simulink model "Ident_friccion_step2_GB3"  (Simulink 6.6)
settings: Solver=ode4  StartTime=0.0  StopTime=1000  RelTol=1e-6
PreLoadFcn:
  | inicializacion_step2
StopFcn:
  | saveDATA_Ident_friccion_STEP2_GB
values from neighbouring files (symbols this model uses):
  k5_id = 0.921382714286    [Valores_identificados_STEP1.mat]
  kb_id = 2.2683494    [Valores_identificados_STEP1.mat]
  Ki1 = 0.0195    [inicializacion_step2.m]
  Ki2 = 0.0195    [inicializacion_step2.m]
  Kp1 = 0.3    [inicializacion_step2.m]
  Kp2 = 0.3    [inicializacion_step2.m]
  precision = precisiones(7)    [inicializacion_step2.m]
  tau1 = 0.008    [inicializacion_step2.m]
  tau_Fs = 0.001    [correccion.m]    (also in inicializacion_step2.m)
  teta1 = 40    [inicializacion_step2.m]
  teta2 = 20    [inicializacion_step2.m]
  zero_c = 100    [inicializacion_step2.m]
  zero_h = 100    [inicializacion_step2.m]
libraries: simulink x7, xpclib x4, xpcnilib x3
settings Model: Creator=CVV  LastModifiedBy=BEJARANO_ROBOT2GDL  SimulationMode=external  ExtModeArmWhenConnect=off  BufferReuse=off
settings DataIOCC: Decimation=5  MaxDataPoints=100000000
settings OptimizationCC: BlockReduction=off  OptimizeBlockIOStorage=off  BufferReuse=off  ExpressionFolding=off  FoldNonRolledExpr=off  LocalBlockOutputs=off
settings DebuggingCC: SignalResolutionControl=TryResolveAllWithWarning  MultiTaskDSMMsg=warning  MultiTaskCondExecSysMsg=none  StrictBusMsg=None
settings RTWCC: SystemTargetFile=xpctarget.tlc  TemplateMakefile=xpc_default_tmf  Description=xPC Target  ProcessScript=xpctarget_make_rtw_hook  IncludeERTFirstTime=on
settings xpcTargetCC: TargetFcnLib=ansi_tfl_tmw.mat  GenFloatMathFcnCalls=ANSI_C  PortableWordSizes=off  RL32LogBufSizeModifier=6000000

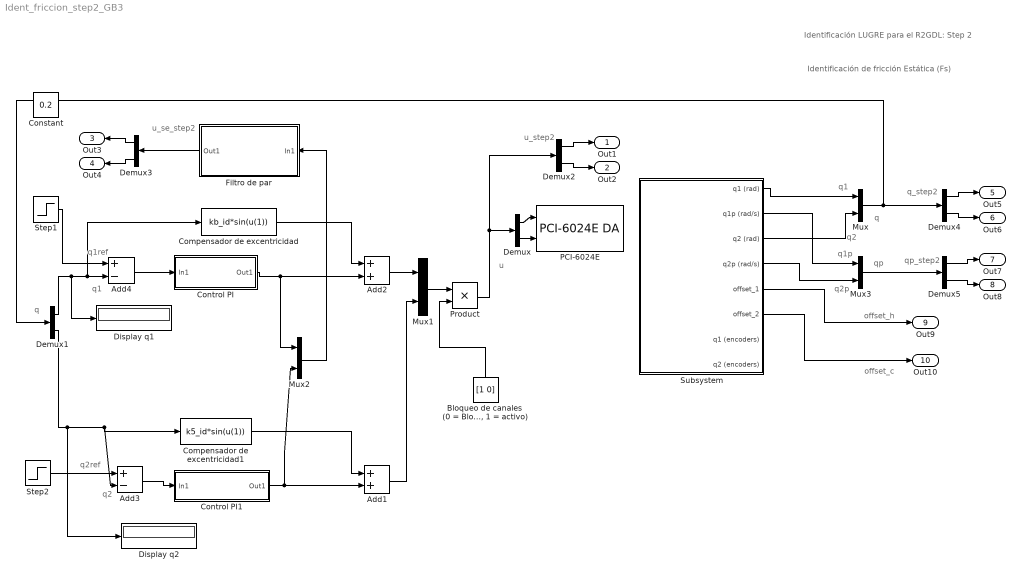
== system Ident_friccion_step2_GB3 ==
  note: Identificación LUGRE para el R2GDL: Step 2
  note: Identificación de fricción Estática (Fs)
  note: q1
  note: q2
  note: q1p
  note: q2p
  note: q
  note: qp
  note: q1
  note: q2
  note: q1ref
  note: q2ref
  note: u
  note: q
  note: u_step2
  note: q_step2
  note: qp_step2
  note: u_se_step2
  note: offset_h
  note: offset_c
  Add1 : Sum  OutScaling=2^-10
  Add2 : Sum  OutScaling=2^-10
  Add3 : Sum  Inputs=+-  OutScaling=2^-10
  Add4 : Sum  Inputs=+-  OutScaling=2^-10
  "Bloqueo de canales  (0 = Bloqueado, 1 = activo)" : Constant  Orientation=up  Value=[1 0]
  Compensador de excentricidad : Fcn  Expr=kb_id*sin(u(1))
  Compensador de excentricidad1 : Fcn  Expr=k5_id*sin(u(1))
  Control PI : Subsystem
  Control PI1 : Subsystem
  Demux{,1..2,4..5} (5 alike) : Demux  Outputs=2
  Demux3 : Demux  Orientation=left  Outputs=2
  Display q1 : Display
  Display q2 : Display
  Filtro de par : Subsystem  Orientation=left
  Mux{,1..3} (4 alike) : Mux  Inputs=2
  "PCI-6024E " : xpcnilib/D//A/PCI-6024E DA  channel=[1,2]  reset=[1]  initValue=[0]  sampletime=0.001  slot=-1
  Product : Product  RndMeth=Zero
  Step1 : Step  Time=0  After=teta1*pi/180  SampleTime=0
  Step2 : Step  Time=0  After=teta2*pi/180  SampleTime=0
  Subsystem : Subsystem
  Out1 : Outport
  Out2 : Outport  Port=2
  Out3 : Outport  Orientation=left  Port=3
  Out4 : Outport  Orientation=left  Port=4
  Out5 : Outport  Port=5
  Out6 : Outport  Port=6
  Out7 : Outport  Port=7
  Out8 : Outport  Port=8
  Out9 : Outport  Port=9
  Out10 : Outport  Port=10
  Constant : Constant  IOType=siggen  Value=0.2
  wires:
  "Bloqueo de canales  (0 = Bloqueado, 1 = activo)"/1 -> Product/2
  Mux1/1 -> Product/1
  Product/1 -> Demux/1, Demux2/1
  Step1/1 -> Add4/1
  Demux1/1 -> Compensador de excentricidad/1, Add4/2, Display q1/1
  Add2/1 -> Mux1/1
  Control PI/1(Out1) -> Add2/2, Mux2/1
  Compensador de excentricidad/1 -> Add2/1
  Add3/1 -> Control PI1/1(In1)
  Demux1/2 -> Compensador de excentricidad1/1, Add3/2, Display q2/1
  Add1/1 -> Mux1/2
  Control PI1/1(Out1) -> Add1/2, Mux2/2
  Compensador de excentricidad1/1 -> Add1/1
  Step2/1 -> Add3/1
  Mux2/1 -> Filtro de par/1(In1)
  Add4/1 -> Control PI/1(In1)
  Demux/2 -> "PCI-6024E "/2
  Demux/1 -> "PCI-6024E "/1
  Subsystem/1(q1 (rad)) -> Mux/1
  Subsystem/2(q1p (rad/s)) -> Mux3/1
  Subsystem/3(q2 (rad)) -> Mux/2
  Subsystem/4(q2p (rad/s)) -> Mux3/2
  Mux/1 -> Demux1/1, Demux4/1
  Mux3/1 -> Demux5/1
  Filtro de par/1(Out1) -> Demux3/1
  Demux2/1 -> Out1/1
  Demux2/2 -> Out2/1
  Demux3/1 -> Out3/1
  Demux3/2 -> Out4/1
  Demux4/2 -> Out6/1
  Demux4/1 -> Out5/1
  Demux5/1 -> Out7/1
  Demux5/2 -> Out8/1
  Subsystem/5(offset_1) -> Out9/1
  Subsystem/6(offset_2) -> Out10/1

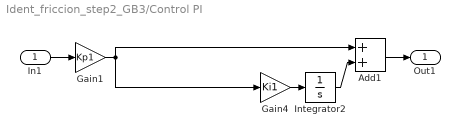
== system Ident_friccion_step2_GB3/Control PI ==
  In1 : Inport
  Add1 : Sum  OutScaling=2^-10
  Gain1 : Gain  Gain=Kp1
  Gain4 : Gain  Gain=Ki1
  Integrator2 : Integrator
  Out1 : Outport
  wires:
  Gain4/1 -> Integrator2/1
  Gain1/1 -> Add1/1, Gain4/1
  Integrator2/1 -> Add1/2
  In1/1 -> Gain1/1
  Add1/1 -> Out1/1

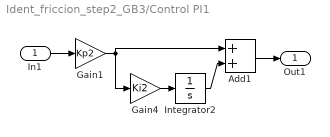
== system Ident_friccion_step2_GB3/Control PI1 ==
  In1 : Inport
  Add1 : Sum  OutScaling=2^-10
  Gain1 : Gain  Gain=Kp2
  Gain4 : Gain  Gain=Ki2
  Integrator2 : Integrator
  Out1 : Outport
  wires:
  Gain4/1 -> Integrator2/1
  Gain1/1 -> Gain4/1, Add1/1
  Integrator2/1 -> Add1/2
  In1/1 -> Gain1/1
  Add1/1 -> Out1/1

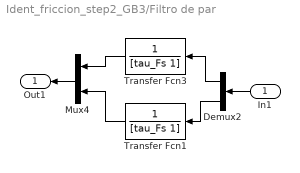
== system Ident_friccion_step2_GB3/Filtro de par ==
  In1 : Inport  Orientation=left
  Demux2 : Demux  Orientation=left  Outputs=2
  Mux4 : Mux  Orientation=left  Inputs=2
  Transfer Fcn1 : TransferFcn  Orientation=left  Denominator=[tau_Fs 1]
  Transfer Fcn3 : TransferFcn  Orientation=left  Denominator=[tau_Fs 1]
  Out1 : Outport  Orientation=left
  wires:
  Demux2/1 -> Transfer Fcn3/1
  Demux2/2 -> Transfer Fcn1/1
  Transfer Fcn3/1 -> Mux4/1
  Transfer Fcn1/1 -> Mux4/2
  Mux4/1 -> Out1/1
  In1/1 -> Demux2/1

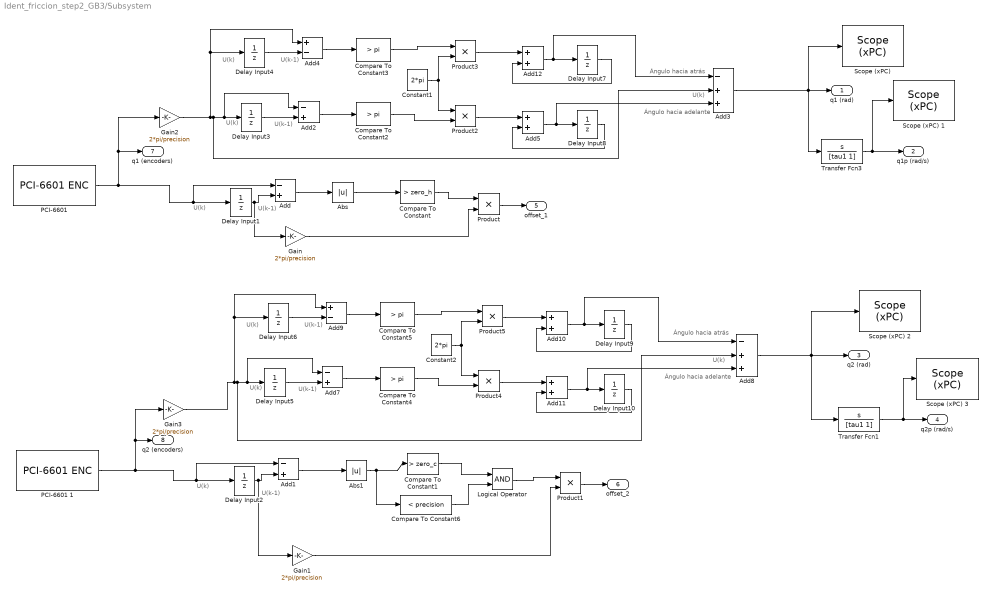
== system Ident_friccion_step2_GB3/Subsystem ==
  note: U(k)
  note: U(k)
  note: U(k-1)
  note: U(k-1)
  note: U(k)
  note: U(k-1)
  note: U(k-1)
  note: U(k)
  note: U(k)
  note: Ángulo hacia atrás
  note: Ángulo hacia adelante
  note: U(k)
  note: U(k-1)
  note: U(k-1)
  note: U(k)
  note: U(k)
  note: Ángulo hacia atrás
  note: Ángulo hacia adelante
  Abs : Abs
  Abs1 : Abs
  Add{,1..2,7} (4 alike) : Sum  Inputs=-+  OutScaling=2^-10
  Add{5,10..12} (4 alike) : Sum  OutScaling=2^-10
  Add3 : Sum  Inputs=-++  OutScaling=2^-10
  Add4 : Sum  Inputs=+-  OutScaling=2^-10
  Add8 : Sum  Inputs=-++  OutScaling=2^-10
  Add9 : Sum  Inputs=+-  OutScaling=2^-10
  Compare To Constant : simulink/Logic and Bit Operations/Compare To Constant  SystemSampleTime=-1  relop=>  const=zero_h  LogicOutDataTypeMode=uint8  ZeroCross=off
  Compare To Constant1 : simulink/Logic and Bit Operations/Compare To Constant  SystemSampleTime=-1  relop=>  const=zero_c  LogicOutDataTypeMode=uint8  ZeroCross=off
  Compare To Constant{2..5} (4 alike) : simulink/Logic and Bit Operations/Compare To Constant  SystemSampleTime=-1  relop=>  const=pi  LogicOutDataTypeMode=uint8  ZeroCross=off
  Compare To Constant6 : simulink/Logic and Bit Operations/Compare To Constant  SystemSampleTime=-1  relop=<  const=precision  LogicOutDataTypeMode=uint8  ZeroCross=off
  Constant1 : Constant  Value=2*pi
  Constant2 : Constant  Value=2*pi
  Delay Input{1..10} (10 alike) : UnitDelay  Description=Store in Global RAM  SampleTime=-1
  Gain{,1..3} (4 alike) : Gain  Gain=2*pi/precision
  Logical Operator : Logic  AllPortsSameDT=off  OutDataTypeMode=Specify via dialog
  "PCI-6601 " : xpcnilib/Incremental Encoder/PCI-6601 ENC  channel=1  countMode=Quadrature Mode X1  initCount=0  reload=on  indexPhase=A high B high  filter=None  sampleTime=0.001  slot=-1
  PCI-6601 1 : xpcnilib/Incremental Encoder/PCI-6601 ENC  channel=2  countMode=Quadrature Mode X1  initCount=0  reload=on  indexPhase=A high B high  filter=None  sampleTime=0.001  slot=-1
  Product{,1..5} (6 alike) : Product  RndMeth=Zero
  "Scope (xPC) " : xpclib/Misc./Scope (xPC)   SystemSampleTime=-1  scopeno=1  scopetype=Target  autostart=on  viewmode=Graphical redraw  formatstr='%15.6f'  grid=on  ylimits=[0,0]  nosamples=250  noprepostsamples=0  interleave=1  triggermode=FreeRun  triggersignal=1  triggerlevel=0.0  triggerslope=Either  triggerscope=1  triggersample=0  filename=data.dat  mode=Lazy  writesize=512  autorestart=off
  Scope (xPC) 1 : xpclib/Misc./Scope (xPC)   SystemSampleTime=-1  scopeno=2  scopetype=Target  autostart=on  viewmode=Graphical redraw  formatstr='%15.6f'  grid=on  ylimits=[0,0]  nosamples=250  noprepostsamples=0  interleave=1  triggermode=FreeRun  triggersignal=1  triggerlevel=0.0  triggerslope=Either  triggerscope=1  triggersample=0  filename=data.dat  mode=Lazy  writesize=512  autorestart=off
  Scope (xPC) 2 : xpclib/Misc./Scope (xPC)   SystemSampleTime=-1  scopeno=3  scopetype=Target  autostart=on  viewmode=Graphical redraw  formatstr='%15.6f'  grid=on  ylimits=[0,0]  nosamples=250  noprepostsamples=0  interleave=1  triggermode=FreeRun  triggersignal=1  triggerlevel=0.0  triggerslope=Either  triggerscope=1  triggersample=0  filename=data.dat  mode=Lazy  writesize=512  autorestart=off
  Scope (xPC) 3 : xpclib/Misc./Scope (xPC)   SystemSampleTime=-1  scopeno=4  scopetype=Target  autostart=on  viewmode=Graphical redraw  formatstr='%15.6f'  grid=on  ylimits=[0,0]  nosamples=250  noprepostsamples=0  interleave=1  triggermode=FreeRun  triggersignal=1  triggerlevel=0.0  triggerslope=Either  triggerscope=1  triggersample=0  filename=data.dat  mode=Lazy  writesize=512  autorestart=off
  Transfer Fcn1 : TransferFcn  Numerator=[1 0]  Denominator=[tau1 1]
  Transfer Fcn3 : TransferFcn  Numerator=[1 0]  Denominator=[tau1 1]
  q1 (rad) : Outport
  q1p (rad/s) : Outport  Port=2
  q2 (rad) : Outport  Port=3
  q2p (rad/s) : Outport  Port=4
  offset_1 : Outport  Port=5
  offset_2 : Outport  Port=6
  q1 (encoders) : Outport  Port=7
  q2 (encoders) : Outport  Port=8
  wires:
  "PCI-6601 "/1 -> Gain2/1, q1 (encoders)/1, Delay Input1/1, Add/1
  Delay Input1/1 -> Add/2, Gain/1
  Compare To Constant/1 -> Product/1
  Gain/1 -> Product/2
  Delay Input2/1 -> Add1/2, Gain1/1
  Gain1/1 -> Product1/2
  PCI-6601 1/1 -> Add1/1, Delay Input2/1, Gain3/1, q2 (encoders)/1
  Product/1 -> offset_1/1
  Product1/1 -> offset_2/1
  Add/1 -> Abs/1
  Abs/1 -> Compare To Constant/1
  Add1/1 -> Abs1/1
  Abs1/1 -> Compare To Constant1/1, Compare To Constant6/1
  Delay Input3/1 -> Add2/2
  Gain2/1 -> Delay Input4/1, Add4/1, Add2/1, Delay Input3/1, Add3/2
  Add2/1 -> Compare To Constant2/1
  Compare To Constant2/1 -> Product2/2
  Transfer Fcn3/1 -> q1p (rad/s)/1, Scope (xPC) 1/1
  Delay Input4/1 -> Add4/2
  Add4/1 -> Compare To Constant3/1
  Compare To Constant3/1 -> Product3/1
  Constant1/1 -> Product3/2, Product2/1
  Add3/1 -> q1 (rad)/1, "Scope (xPC) "/1, Transfer Fcn3/1
  Delay Input5/1 -> Add7/2
  Gain3/1 -> Delay Input6/1, Add9/1, Add7/1, Delay Input5/1, Add8/2
  Add7/1 -> Compare To Constant4/1
  Compare To Constant4/1 -> Product4/2
  Delay Input6/1 -> Add9/2
  Add9/1 -> Compare To Constant5/1
  Compare To Constant5/1 -> Product5/1
  Product5/1 -> Add10/1
  Product4/1 -> Add11/1
  Transfer Fcn1/1 -> q2p (rad/s)/1, Scope (xPC) 3/1
  Add8/1 -> q2 (rad)/1, Scope (xPC) 2/1, Transfer Fcn1/1
  Delay Input7/1 -> Add12/2
  Add12/1 -> Delay Input7/1, Add3/1
  Product3/1 -> Add12/1
  Product2/1 -> Add5/1
  Add5/1 -> Delay Input8/1, Add3/3
  Delay Input8/1 -> Add5/2
  Add10/1 -> Delay Input9/1, Add8/1
  Add11/1 -> Delay Input10/1, Add8/3
  Delay Input10/1 -> Add11/2
  Delay Input9/1 -> Add10/2
  Compare To Constant1/1 -> Logical Operator/1
  Compare To Constant6/1 -> Logical Operator/2
  Logical Operator/1 -> Product1/1
  Constant2/1 -> Product5/2, Product4/1
